simulink model "hisf_0014_Usage_of_transition_paths_passingThroughStates"  (R2018b)
settings: Solver=VariableStepAuto  StartTime=0.0  StopTime=10.0  RelTol=1e-3
model workspace (MAT data in the model file):
  Iei = 0.0219914882836
  converter_data = [0  137.465208994  2.232; 0.1  137.065019157  2.075; 0.2  135.864449646  1.975; 0.3  135.664354728  1.846; 0.4  137.565256453  1.72; 0.5  140.366585312  1.564; 0.6  145.268910814  1.409; 0.7  152.872517717  1.254; 0.8  162.9773111  1.096; 0.81  164.27792807  1.08; 0.82  166.178829795  1.061; 0.83  167.979684062  1.043; 0.84  170.080680706  1.028; 0.85  172.781962105  1.012; 0.86  175.383196045  1.002; 0.87  179.585189333  1.002; 0.88  183.587087703  1.001; 0.89  189.890077635  0.998; 0.9  197.693779455  0.999; 0.92  215.902417037  1.001; 0.94  244.515990379  1.002]
  downtab = [0  5  20  35; 0  5  20  35; 0  5  25  40; 0  5  30  50; 0  30  50  80; 0  30  50  80]
  downth = [0; 5; 40; 50; 90; 100]
  emap = [-40  -44  -49  -53  -57  -61  -65  -70  -74  -78  -82; 215  117  85  66  44  29  10  -2  -13  -22  -32; 245  208  178  148  122  104  85  66  48  33  18; 264  260  241  219  193  167  152  133  119  96  85; 264  279  282  275  260  238  223  208  189  171  152; 267  290  293  297  290  275  260  256  234  212  193; 267  297  305  305  305  301  293  282  267  249  226; 267  301  308  312  319  323  319  316  297  279  253; 267  301  312  319  327  327  327  327  312  293  267; 267  301  312  319  327  334  334  334  319  305  275]
  nevec = [800 1200 1600 2000 2400 2800 3200 3600 4000 4400 4800]
  p0 = 0.07934
  p1 = 0.07934
  thvec = [0; 20; 30; 40; 50; 60; 70; 80; 90; 100]
  uptab = [10  30  50  1000000; 10  30  50  1000000; 15  30  50  1000000; 23  41  60  1000000; 40  70  100  1000000; 40  70  100  1000000]
  upth = [0; 25; 35; 50; 90; 100]
  vehicledata = [3.23; 40; 0.3; 1; 50; 0]
settings Model: Creator=amyyang  LastModifiedBy=amyyang

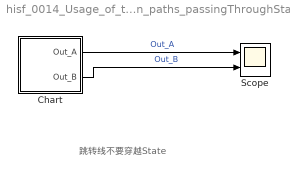
== system hisf_0014_Usage_of_transition_paths_passingThroughStates ==
  note: 跳转线不要穿越State
  Chart : Stateflow chart  TreatAsAtomicUnit=on
  Scope : Scope  NumInputPorts=2
  wires:
  Chart/1(Out_A) -> Scope/1  "Out_A"
  Chart/2(Out_B) -> Scope/2  "Out_B"

== stateflow chart hisf_0014_Usage_of_transition_paths_passingThroughStates/Chart ==
  state A_Parent [parallel]
    en: Out_A = 0;
    settings: executionOrder=1
    state A_sub_2
      du:
      Out_A = Out_A - 1;
    state A_sub_1
      du:
      Out_A = Out_A + 1;
    (default) -> A_sub_1
    A_sub_1 -> A_sub_2 [order 2] : [Out_A==5]
  state B_Parent [parallel]
    en:Out_B = 0;
    settings: executionOrder=2
    state B_sub_2
      du:
      Out_B = Out_B - 1;
    state B_sub_1
      du:
      Out_B = Out_B + 1;
    (default) -> B_sub_1
    B_sub_1 -> B_sub_2 : [Out_B==7]
  note: In the following example, when Out_A is 4, both parent states (A_Parent and
      | B_Parent) are reentered. Reentering the parent states resets the values of Out_A
      | and Out_B to zero.
  A_sub_1 -> B_sub_1 [order 1] : [Out_A == 4]
  data: Out_A output; Out_B output
